simulink model "dc_motor_12v_simscape"  (R2026a)
settings: Solver=ode23t  StopTime=sim_stop_time
model workspace (MAT data in the model file):
  B_load = 0.0001
  J_load = 0.0002
  J_rotor = 1e-05
  K_back_emf_rpm = 0.003
  L_armature = 0.0005
  R_armature = 1.2
  V_supply = 12
  sim_stop_time = 2
  w_initial = 0
libraries: fl_lib x7, nesl_utility x2, ee_lib x1
settings Model: Creator=PattarapolSangaroon  LastModifiedBy=PattarapolSangaroon

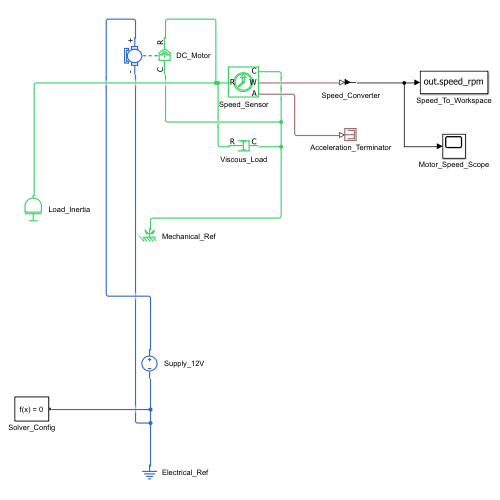
[thumbnail: Simulink's stored preview of the top-level diagram]
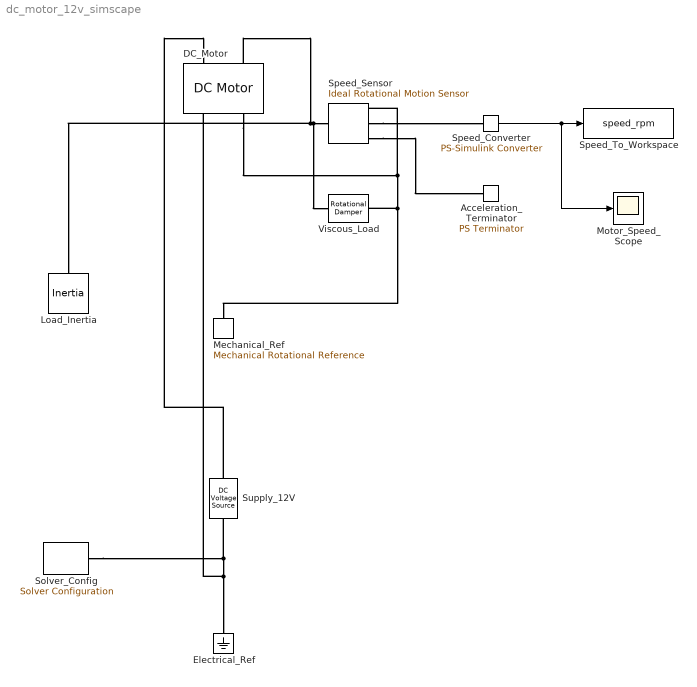
== system dc_motor_12v_simscape ==
  Acceleration_Terminator : fl_lib/Physical Signals/Sinks/PS Terminator
  DC_Motor : ee_lib/Electromechanical/Brushed Motors/DC Motor  field_option=ee.enum.field_option.pm  Rf=100 Ohm  Lf=1 H  Laf=0.15 H  If0=0 A  parameterization=ee.enum.dcparam_option.circuit_param  Ra=R_armature Ohm  La=L_armature H  emf_or_torque=ee.enum.emf_or_torque.kv  Kv=K_back_emf_rpm V/rpm  Ki=6.876e-4 N*m/A  T_stall=0.24e-3 N*m  w_max=19100 rpm  w_rated=15000 rpm  P_rated=0.08 W  V_rated=1.5 V  lam_param=ee.enum.lam_param.damping  i_noload=0 A  V_i_noload=1.5 V  J=J_rotor kg*m^2  lam=0 N*m*s/rad  speed0=0 rpm  alpha=3.93e-3 1/K  Tmeas=25 degC  thermal_mass=100 J/K  initial_temperature=25 degC
  Electrical_Ref : fl_lib/Electrical/Electrical Elements/Electrical Reference
  Load_Inertia : fl_lib/Mechanical/Rotational Elements/Inertia  inertia=J_load kg*m^2  num_ports=foundation.enum.numPorts2.one  w_specify=on  w_priority=High  w=w_initial rad/s  w_nominal_specify=off  w_nominal_value=1  w_nominal_unit=rad/s  t_specify=off  t_priority=None  t=0 N*m  t_nominal_specify=off  t_nominal_value=1  t_nominal_unit=N*m
  Mechanical_Ref : fl_lib/Mechanical/Rotational Elements/Mechanical Rotational Reference
  Motor_Speed_Scope : Scope
  Solver_Config : nesl_utility/Solver Configuration  PhysicalDomain=network_engine_domain  SubClassName=solver  LeftPortType=input  RightPortType=generic  Tones=[]  Harmonics=[]  SimulateNoise=off  Profile=off  UseLocalSampling=off  EnableSwitchedLinearOptims=on  FrequencyDomain=off  UseCCode=off  RelTol=0.001  AbsTol=0.001  MinStep=1e-09  ToWorkspace=off  RevertToSquareIcSolve=off  NumHomotopyIterations=100  PhasorMode=off  PhasorModeNumHarmonics=1  ConsistencySolver=NEWTON_XTOL_AFTER_FTOL  CanonicalOrdering=CANONICAL  OptimizeIntermediates=OPTIMIZED  IndexReductionMethod=DerivativeReplacement  DoDC=off  ResidualTolerance=1e-09  ConsistencyTolSource=GLOBAL  ConsistencyAbsTol=0.001  ConsistencyRelTol=0.001  ConsistencyTolFactor=0.001  UseLocalSolver=off  LocalSolverChoice=NE_BACKWARD_EULER_ADVANCER  ResolveIndetEquations=on  FunctionEvalNumThread=1  LocalSolverSampleTime=0.001  DoFixedCost=off  MaxNonlinIter=3  MaxModeIter=2  ComputeImpulses=off  ImpulseIterations=2  LinearAlgebra=auto  LinearAlgebraNumThread=0  EquationFormulation=NE_TIME_EF  DelaysMemoryBudget=1024  AutomaticFiltering=on  FilteringTimeConstant=0.001  PartitionStorageMethod=AS_NEEDED  PartitionMemoryBudget=1024  PartitionMethod=ROBUST  MultibodyUseLocalSolver=off  MultibodyLocalSolverChoice=ODE1  MultibodyLocalSolverSampleTime=0.001
  Speed_Converter : nesl_utility/PS-Simulink Converter  PhysicalDomain=network_engine_domain  SubClassName=ps_output  LeftPortType=input  RightPortType=output  PseudoPeriodic=off  Frequencies=[]  VectorFormat=inherit  Unit=rpm  AffineConversion=off
  Speed_Sensor : fl_lib/Mechanical/Mechanical Sensors/Ideal Rotational Motion Sensor  reference=foundation.enum.MeasurementReference.difference  acceleration_port=false  velocity_port=true  position_port=true  wrap_angle=false  offset=0 rad
  Speed_To_Workspace : ToWorkspace  VariableName=speed_rpm  SaveFormat=Timeseries  SampleTime=-1
  Supply_12V : fl_lib/Electrical/Electrical Sources/DC Voltage Source  v0=V_supply V
  Viscous_Load : fl_lib/Mechanical/Rotational Elements/Rotational Damper  D=B_load N*m*s/rad  w_specify=off  w_priority=None  w=0 rad/s  w_nominal_specify=off  w_nominal_value=1  w_nominal_unit=rad/s  t_specify=off  t_priority=None  t=0 N*m  t_nominal_specify=off  t_nominal_value=1  t_nominal_unit=N*m
  wires:
  Speed_Converter/1 -> Speed_To_Workspace/1, Motor_Speed_Scope/1
  connections:
  Speed_Sensor/RConn3 -- Acceleration_Terminator/LConn1
  Speed_Sensor/RConn2 -- Speed_Converter/LConn1
  Mechanical_Ref/LConn1 -- Speed_Sensor/RConn1 -- DC_Motor/RConn2 -- Viscous_Load/RConn1
  Speed_Sensor/LConn1 -- DC_Motor/LConn2 -- Load_Inertia/LConn1 -- Viscous_Load/LConn1
  DC_Motor/RConn1 -- Solver_Config/RConn1 -- Supply_12V/RConn1 -- Electrical_Ref/LConn1
  Supply_12V/LConn1 -- DC_Motor/LConn1
